simulink subsystem "Pomieszczenie"  (R2023b)
settings: Solver=VariableStepAuto  StartTime=0.0  StopTime=10.0  RelTol=1e-3
undefined symbols (not defined in the file): cg_2, Cvg2, Cvw2, Kcg2, Kcw2, T_gp0, T_wew0
settings Model: Creator=tomasz  LastModifiedBy=tomasz

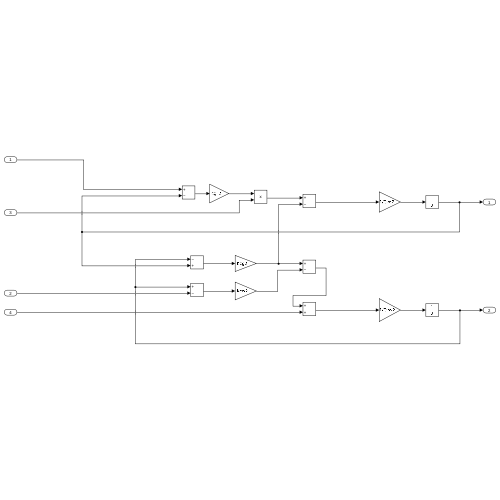
[thumbnail: Simulink's stored preview of the top-level diagram]
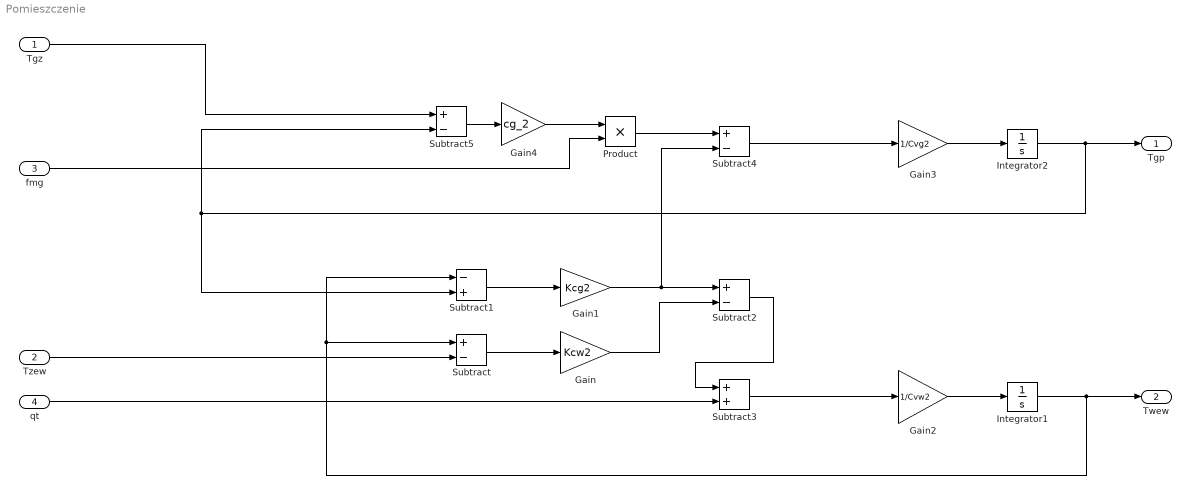
== system Pomieszczenie ==
  Tgz : Inport
  Tzew : Inport  Port=2
  fmg : Inport  Port=3
  qt : Inport  Port=4
  Gain : Gain  Gain=Kcw2
  Gain1 : Gain  Gain=Kcg2
  Gain2 : Gain  Gain=1/Cvw2
  Gain3 : Gain  Gain=1/Cvg2
  Gain4 : Gain  Gain=cg_2
  Integrator1 : Integrator  InitialCondition=T_wew0
  Integrator2 : Integrator  InitialCondition=T_gp0
  Product : Product
  Subtract{,2,4..5} (4 alike) : Sum  Inputs=+-
  Subtract1 : Sum  Inputs=-+
  Subtract3 : Sum
  Tgp : Outport
  Twew : Outport  Port=2
  wires:
  Gain4/1 -> Product/1
  Tzew/1 -> Subtract/2
  Subtract1/1 -> Gain1/1
  Subtract2/1 -> Subtract3/1
  Integrator1/1 -> Twew/1, Subtract/1, Subtract1/1
  Subtract3/1 -> Gain2/1
  Tgz/1 -> Subtract5/1
  Product/1 -> Subtract4/1
  Gain2/1 -> Integrator1/1
  Gain1/1 -> Subtract2/1, Subtract4/2
  Integrator2/1 -> Subtract1/2, Subtract5/2, Tgp/1
  Gain3/1 -> Integrator2/1
  Gain/1 -> Subtract2/2
  qt/1 -> Subtract3/2
  Subtract/1 -> Gain/1
  Subtract5/1 -> Gain4/1
  Subtract4/1 -> Gain3/1
  fmg/1 -> Product/2
